simulink model "simple_compare"  (R2020b)
settings: Solver=VariableStepAuto  StartTime=0.0  StopTime=10.0  RelTol=1e-3
libraries: simulink x2
settings Model: Creator=intel  LastModifiedBy=intel

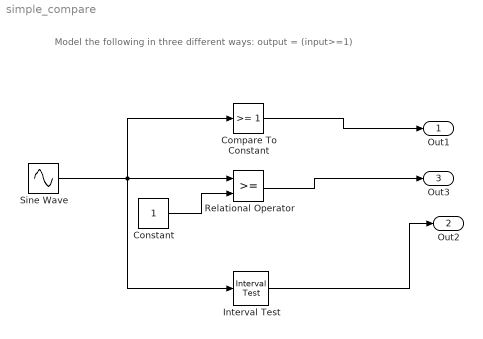
== system simple_compare ==
  note: Model the following in three different ways: output = (input>=1)
  Compare To Constant : simulink/Logic and Bit Operations/Compare To Constant  relop=>=  const=1  OutDataTypeStr=boolean
  Constant : Constant
  Interval Test : simulink/Logic and Bit Operations/Interval Test  IntervalClosedRight=on  uplimit=inf  IntervalClosedLeft=on  lowlimit=1  OutDataTypeStr=boolean
  Relational Operator : RelationalOperator  OutDataTypeStr=boolean  RndMeth=Simplest
  Sine Wave : Sin  SampleTime=0
  Out1 : Outport
  Out2 : Outport  Port=2
  Out3 : Outport  Port=3
  wires:
  Sine Wave/1 -> Interval Test/1, Compare To Constant/1, Relational Operator/1
  Constant/1 -> Relational Operator/2
  Compare To Constant/1 -> Out1/1
  Interval Test/1 -> Out2/1
  Relational Operator/1 -> Out3/1
